simulink model "Simulation_18thJune"  (R2022b)
settings: Solver=VariableStepAuto  StartTime=0.0  StopTime=1.3  RelTol=1e-3
values from neighbouring files (symbols this model uses):
  C_f = 0.000112315*9    (= 0.001010835)    [Main.m]    (also in PSO_2paras.m = swarm(i,2); PSO_filter_2paras.m = swarm(i,2)/10000; Primary_test1.m; Script_18June.m = 0.0112315)
  f_c = 50e3    (= 50000)    [Main.m]    (also in Primary_test1.m; Script_18June.m; Script_23June.m; Script_5thJune.m)
  k = -0.5    [Main.m]    (also in Primary_test1.m; Savedata.m = 0.2909; Script_18June.m = 0.5; Script_23June.m)
  K_h11 = 0    [Main.m]    (also in PSO_HC.m = swarm(i,4); Primary_test1.m; Script_18June.m; Script_23June.m)
  K_h13 = 0    [Main.m]    (also in Primary_test1.m; Script_18June.m; Script_23June.m; Script_5thJune.m)
  K_h5 = 0    [Main.m]    (also in PSO_HC.m = swarm(i,1); Primary_test1.m = 1; Script_18June.m; Script_23June.m)
  K_h7 = 0    [Main.m]    (also in PSO_HC.m = swarm(i,2); Primary_test1.m; Script_18June.m; Script_23June.m)
  K_h9 = 0    [Main.m]    (also in PSO_HC.m = swarm(i,3); Script_18June.m; Script_23June.m; Script_5thJune.m)
  ki_pr = 160    [Main.m]    (also in PSO.m = swarm(i,2); Primary_test1.m; Savedata.m = 422.4716; Script_18June.m = 150)
  kL = 1e-7    (= 1e-07)    [Main.m]    (also in Primary_test1.m; Script_18June.m; Script_23June.m; Script_5thJune.m)
  Kp_pr = 1.7    [Main.m]    (also in PSO.m = swarm(i,1); Primary_test1.m; Savedata.m = 0.9028; Script_18June.m = 1)
  L_f = 0.000659829*1.4    (= 0.0009237606)    [Main.m]    (also in PSO_2paras.m = swarm(i,1); PSO_filter_2paras.m = swarm(i,1); Primary_test1.m; Script_18June.m = 0.000295603392)
  L_in1 = 0.35e-3    (= 0.00035)    [Main.m]    (also in Primary_test1.m; Script_18June.m; Script_23June.m; Script_5thJune.m)
  L_in2 = 0.35e-3    (= 0.00035)    [Main.m]    (also in Primary_test1.m; Script_18June.m; Script_23June.m; Script_5thJune.m)
  LD_ref1 = 100e-6    (= 0.0001)    [Main.m]    (also in Primary_test1.m; Script_18June.m = 5e-05; Script_23June.m = 1e-05; Script_5thJune.m = 1e-05)
  lo_co = 0.1    [Main.m]    (also in Primary_test1.m; Script_18June.m; Script_23June.m; Script_5thJune.m)
  load_off = 28    [Main.m]    (also in Primary_test1.m = 2; Script_18June.m; Script_23June.m; Script_5thJune.m = 10)
  load_on = 0.21    [Main.m]    (also in Primary_test1.m = 1; Script_18June.m; Script_23June.m; Script_5thJune.m)
  m_p1 = 9.4e-5/droopDivide    (= 9.4e-06)    [Main.m]    (also in Primary_test1.m; Script_18June.m = 9.4e-05; Script_23June.m = 9.4e-05; Script_5thJune.m = 5e-05)
  m_p2 = 9.4e-5/droopDivide    (= 9.4e-06)    [Main.m]    (also in Primary_test1.m; Script_18June.m = 9.4e-05; Script_23June.m = 9.4e-05; Script_5thJune.m = 5e-05)
  m_p3 = 11.4e-5/droopDivide    (= 1.14e-05)    [Main.m]    (also in Primary_test1.m; Script_18June.m = 0.000114; Script_23June.m = 0.000114; Script_5thJune.m = 6.42857142857e-05)
  m_p4 = 11.4e-5/droopDivide    (= 1.14e-05)    [Main.m]    (also in Primary_test1.m; Script_18June.m = 0.000114; Script_23June.m = 0.000114; Script_5thJune.m = 6.42857142857e-05)
  n_q1 = 1.3e-3/droopDivide2    (= 6.5e-05)    [Main.m]    (also in Primary_test1.m; Script_18June.m; Script_23June.m; Script_5thJune.m = 0.2)
  n_q2 = 1.3e-3/droopDivide2    (= 6.5e-05)    [Main.m]    (also in Primary_test1.m; Script_18June.m; Script_23June.m; Script_5thJune.m = 0.2)
  n_q3 = 1.5e-3/droopDivide2    (= 7.5e-05)    [Main.m]    (also in Primary_test1.m; Script_18June.m; Script_23June.m; Script_5thJune.m = 0.257142857143)
  n_q4 = 1.5e-3/droopDivide2    (= 7.5e-05)    [Main.m]    (also in Primary_test1.m; Script_18June.m; Script_23June.m; Script_5thJune.m = 0.257142857143)
  PMW = V_nom/0.55    [Main.m]    (also in Primary_test1.m; Script_18June.m = V_nom/0.4; Script_23June.m; Script_5thJune.m = 220*sqrt(2))
  R_f = 0.35    [Main.m]    (also in PSO_filter_2paras.m = 10*L_f; Primary_test1.m; Savedata.m = 0.249593207053; Script_18June.m = 0.1)
  R_in1 = 0.03    [Main.m]    (also in Primary_test1.m; Script_18June.m; Script_23June.m; Script_5thJune.m)
  R_in2 = 0.03    [Main.m]    (also in Primary_test1.m; Script_18June.m; Script_23June.m; Script_5thJune.m)
  Ts = 10e-6    (= 1e-05)    [Main.m]    (also in Primary_test1.m; Script_18June.m; Script_23June.m; Script_5thJune.m)
  V_nom = 220*sqrt(2)    [Main.m]    (also in Primary_test1.m; Script_18June.m; Script_23June.m; Script_5thJune.m)
  Vdc = 600    [Main.m]    (also in Primary_test1.m; Script_18June.m; Script_23June.m; Script_5thJune.m)
  w_c_high = 2*pi*50    (= 314.159265359)    [Main.m]    (also in Primary_test1.m; Script_18June.m = 307.876080052; Script_23June.m; Script_5thJune.m = 307.876080052)
  w_nom = 2*pi*f    (= 314.159265359)    [Main.m]    (also in Primary_test1.m; Script_18June.m; Script_23June.m; Script_5thJune.m)
  wc_hc = 1    [Main.m]    (also in Primary_test1.m; Script_18June.m = 0.3; Script_23June.m; Script_5thJune.m = 0.3)
  wc_pr = 3    [Main.m]    (also in PSO.m = swarm(i,3); Primary_test1.m; Savedata.m = 1.36672; Script_18June.m = 1.5)
undefined symbols (not defined in the file or in its folder): i
libraries: eeGeneralControl x16, spsThreePhaseSeriesRLCBranchLib x15, spsThreePhaseVIMeasurementLib x12, spsabctodq0Lib x12, slpidlib x8, spsThreePhaseSeriesRLCLoadLib x5, spsThreePhaseBreakerLib x5, spsDCVoltageSourceLib x5, spsSeriesRLCBranchLib x5, spsTriangleGeneratorLib x4, spsTwoLevelConverterLib x4, spsIGBTLib x2
(part 3 of 4)

== system Simulation_18thJune/Voltage Source Inverter 2/PLL_1p2 ==
  v : Inport
  2pi : Constant  Value=2*pi
  Low-Pass Filter (Discrete or Continuous) : eeGeneralControl/Low-Pass Filter (Discrete or Continuous)  K=1  T=lo_co  B=inf  A=-inf  init_option=Inherited from block input  x0=0  Ts=-1
  PID Controller : slpidlib/PID Controller  Controller=PI  Form=Parallel  TimeDomain=Continuous-time  UseExternalTs=off  SampleTime=-1  IntegratorMethod=Forward Euler  FilterMethod=Forward Euler  ControllerParametersSource=internal  P=100.15925  I=9869  UseKiTs=off  D=0  N=100  UseFilter=on  TunerSelectOption=Transfer Function Based (PID Tuner App)  InitialConditionSource=internal  InitialConditionForIntegrator=0  InitialConditionForFilter=0  DifferentiatorICPrevScaledInput=0  ExternalReset=none  TrackingMode=off  Kt=1  LimitOutput=off  SatLimitsSource=internal  UpperSaturationLimit=inf  LowerSaturationLimit=-inf  LinearizeAsGain=off  AntiWindupMode=none  Kb=1  LimitIntegrator=off  UpperIntegratorSaturationLimit=inf  LowerIntegratorSaturationLimit=-inf  POutMin=[]  POutMax=[]  IOutMin=[]  IOutMax=[]  DOutMin=[]  DOutMax=[]  NOutMin=[]  NOutMax=[]  SumOutMin=[]  SumOutMax=[]  SaturationOutMin=[]  SaturationOutMax=[]  PParamMin=[]  PParamMax=[]  IParamMin=[]  IParamMax=[]  DParamMin=[]  DParamMax=[]  NParamMin=[]  NParamMax=[]  KbParamMin=[]  KbParamMax=[]  KtParamMin=[]  KtParamMax=[]  KbOutMin=[]  KbOutMax=[]  KtOutMin=[]  KtOutMax=[]  IntegratorOutMin=[]  IntegratorOutMax=[]  FilterOutMin=[]  FilterOutMax=[]  SumI1OutMin=[]  SumI1OutMax=[]  SumI2OutMin=[]  SumI2OutMax=[]  SumI3OutMin=[]  SumI3OutMax=[]  SumI4OutMin=[]  SumI4OutMax=[]  SumDOutMin=[]  SumDOutMax=[]  DifferentiatorOutMin=[]  DifferentiatorOutMax=[]  FilterDiffOutCoefMin=[]  FilterDiffOutCoefMax=[]  ReciprocalOutMin=[]  ReciprocalOutMax=[]  SumDenOutMin=[]  SumDenOutMax=[]  SumNumOutMin=[]  SumNumOutMax=[]  DivideOutMin=[]  DivideOutMax=[]  UdiffTsProdOutMin=[]  UdiffTsProdOutMax=[]  NTsProdOutMin=[]  NTsProdOutMax=[]  UintegralTsProdOutMin=[]  UintegralTsProdOutMax=[]  UngainTsProdOutMin=[]  UngainTsProdOutMax=[]  ClampingZeroOutDataTypeStr=Inherit: Inherit via back propagation  ClampingZeroOutMin=[]  ClampingZeroOutMax=[]  FilterDenConstantOutDataTypeStr=Inherit: Inherit via back propagation  FilterDenConstantOutMin=[]  FilterDenConstantOutMax=[]  PCopyOutDataTypeStr=Inherit: Inherit via back propagation  PCopyOutMin=[]  PCopyOutMax=[]  NCopyOutDataTypeStr=Inherit: Inherit via back propagation  NCopyOutMin=[]  NCopyOutMax=[]  IntegratorContinuousStateAttributes=''  IntegratorStateMustResolveToSignalObject=off  IntegratorRTWStateStorageClass=Auto  FilterContinuousStateAttributes=''  FilterStateMustResolveToSignalObject=off  FilterRTWStateStorageClass=Auto  ParallelPVariant=InternalParameters  IdealPVariant=Disabled  IVariant=InternalParameters  DVariant=Disabled  IntegratorVariant=Continuous  SatVariant=Disabled  AWVariant=Passthrough  PCopyVariant=Disabled  TRVariant=Disabled  FdbkBlocksVariant=Forward  IdealPFdbkVariant=Disabled  SatFdbkVariant=Disabled  DerivativeFilterVariant=Disabled  NVariant=Disabled  NCopyVariant=Disabled_SignalSpec  FilterICVariant=Disabled  IntegratorICVariant=InternalICs  ExternalResetVariant=Disabled  TRSumVariant=Passthrough  SumFdbkVariant=Disabled  SumVariant=Sum_PI  TsampFilterVariant=InternalTs  TsampNgainVariant=Passthrough  TsampIntegralVariant=Passthrough  ExternalSaturationOutDataTypeStr=Inherit: Same as second input
  Reset1 : RelationalOperator  OutDataTypeStr=boolean  InputSameDT=off
  Scope : Scope
  Sqrt : Sqrt
  Square : Math  Operator=square
  Square1 : Math  Operator=square
  Sum : Sum  Inputs=|++
  Sum1 : Sum  Inputs=|++
  TienXuly : Subsystem  mask{k=0.5, fc1=50, fc2=10}
      mask prompts: k "he so k"; fc1 "Tan so cat cua bo loc bac 2"; fc2 "Tan so cat cua bo loc thong thap"
  Tinhtheta : Integrator  ExternalReset=rising  UpperSaturationLimit=2*pi
  apha-beta=>dq : Subsystem
  wff : Constant  Value=50*2*pi
  v_dq : Outport
  omega : Outport  Port=2
  wires:
  PID Controller/1 -> Sum1/1
  v/1 -> TienXuly/1(v)
  Tinhtheta/1 -> apha-beta=>dq/1(Theta), Reset1/1
  TienXuly/2(v'q) -> apha-beta=>dq/3(Ubeta)
  apha-beta=>dq/1(vq) -> Square1/1, PID Controller/1
  TienXuly/1(v') -> apha-beta=>dq/2(Uapha)
  2pi/1 -> Reset1/2
  wff/1 -> Sum1/2
  Reset1/1 -> Tinhtheta/2
  apha-beta=>dq/2(vd) -> Square/1
  Square/1 -> Sum/1
  Square1/1 -> Sum/2
  Sum/1 -> Sqrt/1
  Sqrt/1 -> v_dq/1
  Sum1/1 -> Low-Pass Filter (Discrete or Continuous)/1, Tinhtheta/1  "P"
  Low-Pass Filter (Discrete or Continuous)/1 -> Scope/1, omega/1  "P"

== system Simulation_18thJune/Voltage Source Inverter 2/PMW ==
  REF : Inport
  Tri_signal : Inport  Port=2
  Demux : Demux  Outputs=3
  Mux : Mux  Inputs=6
  NOT : Logic  Operator=NOT  AllPortsSameDT=off  OutDataTypeStr=boolean
  NOT1 : Logic  Operator=NOT  AllPortsSameDT=off  OutDataTypeStr=boolean
  NOT2 : Logic  Operator=NOT  AllPortsSameDT=off  OutDataTypeStr=boolean
  Relational Operator : RelationalOperator  OutDataTypeStr=boolean  RndMeth=Simplest  InputSameDT=off
  Relational Operator1 : RelationalOperator  OutDataTypeStr=boolean  RndMeth=Simplest  InputSameDT=off
  Relational Operator2 : RelationalOperator  OutDataTypeStr=boolean  RndMeth=Simplest  InputSameDT=off
  Scope : Scope
  Scope1 : Scope
  Scope2 : Scope  NumInputPorts=2
  Out1 : Outport
  wires:
  Demux/1 -> Relational Operator/1
  Tri_signal/1 -> Relational Operator1/2, Relational Operator/2, Relational Operator2/2
  Demux/2 -> Relational Operator1/1
  Demux/3 -> Relational Operator2/1
  REF/1 -> Scope1/1, Demux/1
  Relational Operator/1 -> Scope2/1, Mux/1, NOT/1
  NOT/1 -> Scope2/2, Mux/2
  Relational Operator1/1 -> NOT1/1, Mux/3
  NOT1/1 -> Mux/4
  Relational Operator2/1 -> Mux/5, NOT2/1
  NOT2/1 -> Mux/6
  Mux/1 -> Scope/1, Out1/1

== system Simulation_18thJune/Voltage Source Inverter 2/PQ calculator ==
  Vod : Inport
  Voq : Inport  Port=2
  Iod : Inport  Port=3
  Ioq : Inport  Port=4
  Product{,1..3} (4 alike) : Product
  Scope : Scope
  Sum10 : Sum  Inputs=|++
  Sum11 : Sum  Inputs=|+-
  p_hat : Outport
  q_hat : Outport  Port=2
  wires:
  Product3/1 -> Sum11/2
  Product1/1 -> Sum10/2
  Voq/1 -> Product3/1, Product1/1
  Iod/1 -> Product/2, Product3/2
  Product2/1 -> Sum11/1
  Ioq/1 -> Product1/2, Product2/2
  Product/1 -> Sum10/1
  Vod/1 -> Scope/1, Product/1, Product2/1
  Sum11/1 -> q_hat/1  "q_hat"
  Sum10/1 -> p_hat/1  "p_hat"

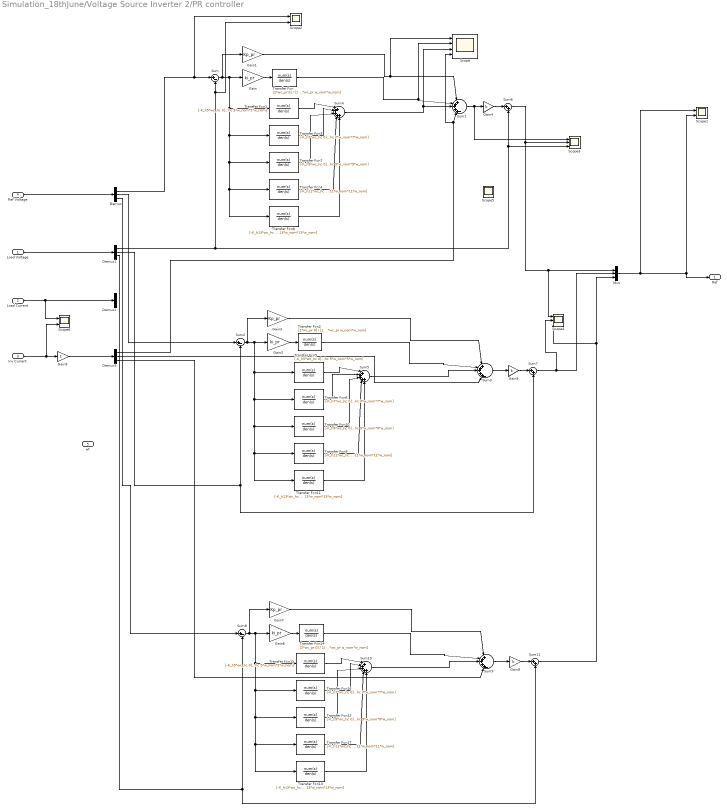
== system Simulation_18thJune/Voltage Source Inverter 2/PR controller ==
  Load Voltage : Inport
  Load Current : Inport  Port=2
  Inv Current : Inport  Port=3
  Ref Voltage : Inport  Port=4
  wt : Inport  Port=5
  Demux{,1..3} (4 alike) : Demux  Outputs=3
  Gain : Gain  Gain=ki_pr
  Gain1 : Gain  Gain=Kp_pr
  Gain2 : Gain  Gain=ki_pr
  Gain3 : Gain  Gain=Kp_pr
  Gain4 : Gain  Gain=k
  Gain5 : Gain  Gain=k
  Gain6 : Gain  Gain=ki_pr
  Gain7 : Gain  Gain=Kp_pr
  Gain8 : Gain  Gain=k
  Gain9 : Gain
  Mux : Mux  Inputs=3
  Scope : Scope  NumInputPorts=4
  Scope{1..2,5..6} (4 alike) : Scope  NumInputPorts=2
  Scope3 : Scope  NumInputPorts=3
  Scope4 : Scope  NumInputPorts=3
  Sum : Sum  Inputs=|+-
  Sum1 : Sum  Inputs=|+++++-
  Sum10 : Sum  Inputs=|+++++
  Sum11 : Sum  Inputs=|++
  Sum2 : Sum  Inputs=|+-
  Sum3 : Sum  Inputs=|+++++-
  Sum4 : Sum  Inputs=|+++++
  Sum5 : Sum  Inputs=|+++++
  Sum6 : Sum  Inputs=|++
  Sum7 : Sum  Inputs=|++
  Sum8 : Sum  Inputs=|+-
  Sum9 : Sum  Inputs=|+++++-
  Transfer Fcn : TransferFcn  Numerator=[2*wc_pr 0]  Denominator=[1 2*wc_pr*wc_pr w_nom*w_nom]
  Transfer Fcn1 : TransferFcn  Numerator=[-K_h5*wc_hc 0]  Denominator=[1 2*wc_hc 5*w_nom*5*w_nom]
  Transfer Fcn10 : TransferFcn  Numerator=[-K_h9*wc_hc 0]  Denominator=[1 2*wc_hc 9*w_nom*9*w_nom]
  Transfer Fcn11 : TransferFcn  Numerator=[-K_h13*wc_hc 0]  Denominator=[1 2*wc_hc 13*w_nom*13*w_nom]
  Transfer Fcn12 : TransferFcn  Numerator=[-K_h9*wc_hc 0]  Denominator=[1 2*wc_hc 9*w_nom*9*w_nom]
  Transfer Fcn13 : TransferFcn  Numerator=[-K_h13*wc_hc 0]  Denominator=[1 2*wc_hc 13*w_nom*13*w_nom]
  Transfer Fcn14 : TransferFcn  Numerator=[2*wc_pr 0]  Denominator=[1 2*wc_pr*wc_pr w_nom*w_nom]
  Transfer Fcn15 : TransferFcn  Numerator=[-K_h5*wc_hc 0]  Denominator=[1 2*wc_hc 5*w_nom*5*w_nom]
  Transfer Fcn16 : TransferFcn  Numerator=[-K_h7*wc_hc 0]  Denominator=[1 2*wc_hc 7*w_nom*7*w_nom]
  Transfer Fcn17 : TransferFcn  Numerator=[-K_h11*wc_hc 0]  Denominator=[1 2*wc_hc 11*w_nom*11*w_nom]
  Transfer Fcn2 : TransferFcn  Numerator=[2*wc_pr 0]  Denominator=[1 2*wc_pr*wc_pr w_nom*w_nom]
  Transfer Fcn3 : TransferFcn  Numerator=[-K_h7*wc_hc 0]  Denominator=[1 2*wc_hc 7*w_nom*7*w_nom]
  Transfer Fcn4 : TransferFcn  Numerator=[-K_h11*wc_hc 0]  Denominator=[1 2*wc_hc 11*w_nom*11*w_nom]
  Transfer Fcn5 : TransferFcn  Numerator=[-K_h5*wc_hc 0]  Denominator=[1 2*wc_hc 5*w_nom*5*w_nom]
  Transfer Fcn6 : TransferFcn  Numerator=[-K_h7*wc_hc 0]  Denominator=[1 2*wc_hc 7*w_nom*7*w_nom]
  Transfer Fcn7 : TransferFcn  Numerator=[-K_h9*wc_hc 0]  Denominator=[1 2*wc_hc 9*w_nom*9*w_nom]
  Transfer Fcn8 : TransferFcn  Numerator=[-K_h13*wc_hc 0]  Denominator=[1 2*wc_hc 13*w_nom*13*w_nom]
  Transfer Fcn9 : TransferFcn  Numerator=[-K_h11*wc_hc 0]  Denominator=[1 2*wc_hc 11*w_nom*11*w_nom]
  Ref : Outport
  wires:
  Ref Voltage/1 -> Demux/1
  Sum/1 -> Gain1/1, Transfer Fcn8/1, Transfer Fcn4/1, Transfer Fcn7/1, Transfer Fcn3/1, Transfer Fcn1/1, Gain/1
  Gain/1 -> Transfer Fcn/1
  Gain1/1 -> Scope/1, Sum1/1
  Transfer Fcn/1 -> Scope/2, Sum1/2
  Mux/1 -> Ref/1, Scope1/2, Scope1/1
  Sum4/1 -> Scope/3, Sum1/3
  Transfer Fcn1/1 -> Sum4/1
  Transfer Fcn3/1 -> Sum4/2
  Transfer Fcn7/1 -> Sum4/3
  Transfer Fcn4/1 -> Sum4/4
  Transfer Fcn8/1 -> Sum4/5
  Load Voltage/1 -> Demux1/1
  Inv Current/1 -> Scope6/2, Gain9/1
  Demux/1 -> Scope2/1, Sum/1
  Demux1/1 -> Sum6/2, Scope3/3, Scope2/2, Sum/2
  Demux3/1 -> Scope/4, Sum1/5
  Sum1/1 -> Scope3/1, Gain4/1
  Gain4/1 -> Sum6/1
  Sum6/1 -> Scope4/1, Mux/1, Scope3/2
  Demux1/2 -> Sum7/2, Sum2/2
  Transfer Fcn9/1 -> Sum5/4
  Sum5/1 -> Sum3/3
  Transfer Fcn6/1 -> Sum5/2
  Transfer Fcn5/1 -> Sum5/1
  Transfer Fcn11/1 -> Sum5/5
  Transfer Fcn10/1 -> Sum5/3
  Gain5/1 -> Sum7/1
  Gain3/1 -> Sum3/1
  Demux/2 -> Sum2/1
  Sum3/1 -> Gain5/1
  Sum2/1 -> Gain3/1, Transfer Fcn11/1, Transfer Fcn9/1, Transfer Fcn10/1, Transfer Fcn6/1, Transfer Fcn5/1, Gain2/1
  Transfer Fcn2/1 -> Sum3/2
  Gain2/1 -> Transfer Fcn2/1
  Sum7/1 -> Scope4/2, Mux/2
  Demux1/3 -> Sum11/2, Sum8/2
  Gain6/1 -> Transfer Fcn14/1
  Sum8/1 -> Gain7/1, Transfer Fcn13/1, Transfer Fcn17/1, Transfer Fcn12/1, Transfer Fcn16/1, Transfer Fcn15/1, Gain6/1
  Gain8/1 -> Sum11/1
  Sum9/1 -> Gain8/1
  Transfer Fcn13/1 -> Sum10/5
  Transfer Fcn12/1 -> Sum10/3
  Gain7/1 -> Sum9/1
  Transfer Fcn15/1 -> Sum10/1
  Transfer Fcn16/1 -> Sum10/2
  Transfer Fcn17/1 -> Sum10/4
  Sum11/1 -> Scope4/3, Mux/3
  Sum10/1 -> Sum9/3
  Demux/3 -> Sum8/1
  Transfer Fcn14/1 -> Sum9/2
  Demux3/2 -> Sum3/5
  Demux3/3 -> Sum9/5
  Load Current/1 -> Scope6/1, Demux2/1
  Gain9/1 -> Demux3/1

== system Simulation_18thJune/Voltage Source Inverter 2/THD measurement ==
  In1 : Inport
  Demux : Demux  Outputs=3
  To Workspace : ToWorkspace  VariableName=phase1  SaveFormat=Structure With Time  SampleTime=-1
  To Workspace1 : ToWorkspace  VariableName=phase2  SaveFormat=Structure With Time  SampleTime=-1
  To Workspace2 : ToWorkspace  VariableName=phase3  SaveFormat=Structure With Time  SampleTime=-1
  wires:
  In1/1 -> Demux/1
  Demux/1 -> To Workspace/1
  Demux/2 -> To Workspace1/1
  Demux/3 -> To Workspace2/1

== system Simulation_18thJune/Voltage Source Inverter 2/dq converter ==
  Vodq : Inport
  Iodq : Inport  Port=2
  Ildq : Inport  Port=3
  wt : Inport  Port=4
  Scope : Scope
  Scope1 : Scope
  Subsystem : Subsystem
  Subsystem1 : Subsystem
  Subsystem2 : Subsystem
  Vod : Outport
  Voq : Outport  Port=2
  Iod : Outport  Port=3
  Ioq : Outport  Port=4
  Ild : Outport  Port=5
  Ilq : Outport  Port=6
  wires:
  Subsystem/1(Out1) -> Scope/1, Vod/1  "Vod"
  Subsystem1/1(Out1) -> Iod/1  "Iod"
  Subsystem/2(Out2) -> Voq/1  "Voq"
  wt/1 -> Subsystem2/2(wt), Subsystem1/2(wt), Subsystem/2(wt)
  Subsystem1/2(Out2) -> Ioq/1  "Ioq"
  Iodq/1 -> Subsystem1/1(abc)
  Subsystem2/2(Out2) -> Ilq/1  "Ilq"
  Ildq/1 -> Subsystem2/1(abc)
  Vodq/1 -> Subsystem/1(abc)
  Subsystem2/1(Out1) -> Scope1/1, Ild/1  "Vod"

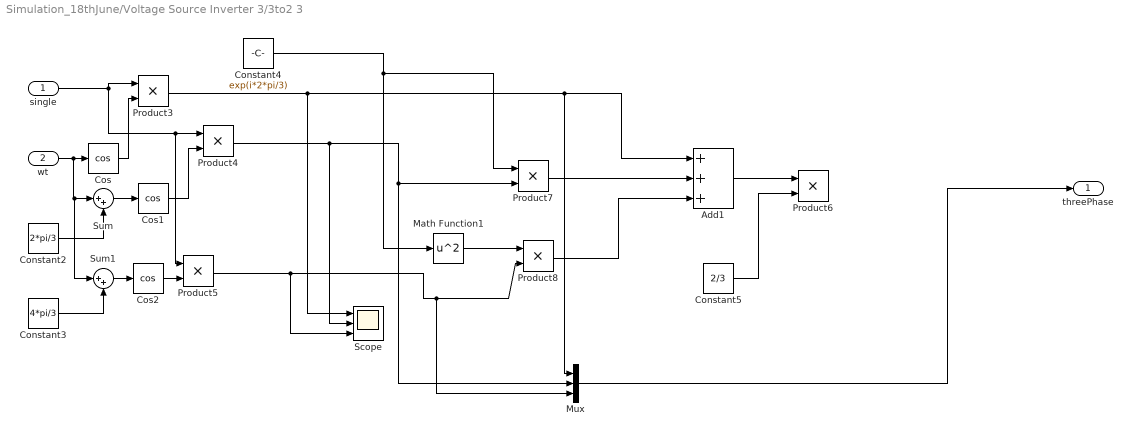
== system Simulation_18thJune/Voltage Source Inverter 3/3to2 3 ==
  "single " : Inport
  "wt " : Inport  Port=2
  Add1 : Sum  Inputs=+++
  Constant2 : Constant  Value=2*pi/3
  Constant3 : Constant  Value=4*pi/3
  Constant4 : Constant  Value=exp(i*2*pi/3)
  Constant5 : Constant  Value=2/3
  Cos : Trigonometry  Operator=cos
  Cos1 : Trigonometry  Operator=cos
  Cos2 : Trigonometry  Operator=cos
  Math Function1 : Math  Operator=square  SignedPower=on
  Mux : Mux  Inputs=3
  Product{3..8} (6 alike) : Product  RndMeth=Zero
  Scope : Scope  NumInputPorts=3
  Sum : Sum  Inputs=|++
  Sum1 : Sum  Inputs=|++
  threePhase : Outport  VectorParamsAs1DForOutWhenUnconnected=off
  wires:
  "single "/1 -> Product5/1, Product4/1, Product3/1
  Cos/1 -> Product3/2
  Constant2/1 -> Sum/2
  Sum/1 -> Cos1/1
  Cos1/1 -> Product4/2
  "wt "/1 -> Sum1/1, Sum/1, Cos/1
  Constant3/1 -> Sum1/2
  Sum1/1 -> Cos2/1
  Cos2/1 -> Product5/2
  Constant4/1 -> Product7/1, Math Function1/1
  Product7/1 -> Add1/2
  Add1/1 -> Product6/1
  Product8/1 -> Add1/3
  Product5/1 -> Scope/3, Mux/3, Product8/2
  Product3/1 -> Scope/1, Mux/1, Add1/1
  Constant5/1 -> Product6/2
  Product4/1 -> Scope/2, Mux/2, Product7/2
  Math Function1/1 -> Product8/1
  Mux/1 -> threePhase/1

== system Simulation_18thJune/Voltage Source Inverter 3/Droop for secondary control2 ==
  P : Inport
  w_nom : Inport  Port=2
  V_nom : Inport  Port=3
  Q : Inport  Port=4
  Gain4 : Gain  Gain=n_q
  Gain5 : Gain  Gain=m_p
  Integrator : Integrator  WrapState=on  WrappedStateUpperValue=2*pi  WrappedStateLowerValue=0
  Sum1 : Sum  Inputs=|+-
  Sum2 : Sum  Inputs=|+-
  Vref : Outport
  wt : Outport  Port=2
  wo : Outport  Port=3
  wires:
  P/1 -> Gain5/1
  w_nom/1 -> Sum2/1
  Gain5/1 -> Sum2/2
  Sum2/1 -> wo/1, Integrator/1  "w"
  Integrator/1 -> wt/1
  V_nom/1 -> Sum1/1  "Vod_s"
  Gain4/1 -> Sum1/2
  Q/1 -> Gain4/1
  Sum1/1 -> Vref/1  "Vod_s"

== system Simulation_18thJune/Voltage Source Inverter 3/Low-pass filter ==
  p_hat : Inport
  q_hat : Inport  Port=2
  Low-Pass Filter (Discrete or Continuous) : eeGeneralControl/Low-Pass Filter (Discrete or Continuous)  K=1  T=lo_co  B=inf  A=-inf  init_option=Inherited from block input  x0=0  Ts=-1
  Low-Pass Filter (Discrete or Continuous)1 : eeGeneralControl/Low-Pass Filter (Discrete or Continuous)  K=1  T=lo_co  B=inf  A=-inf  init_option=Inherited from block input  x0=0  Ts=-1
  P : Outport
  Q : Outport  Port=2
  wires:
  q_hat/1 -> Low-Pass Filter (Discrete or Continuous)1/1
  Low-Pass Filter (Discrete or Continuous)1/1 -> Q/1  "Q"
  Low-Pass Filter (Discrete or Continuous)/1 -> P/1  "P"
  p_hat/1 -> Low-Pass Filter (Discrete or Continuous)/1

== system Simulation_18thJune/Voltage Source Inverter 3/PLL_1p1 ==
  v : Inport
  2pi : Constant  Value=2*pi
  Low-Pass Filter (Discrete or Continuous) : eeGeneralControl/Low-Pass Filter (Discrete or Continuous)  K=1  T=lo_co  B=inf  A=-inf  init_option=Inherited from block input  x0=0  Ts=-1
  PID Controller : slpidlib/PID Controller  Controller=PI  Form=Parallel  TimeDomain=Continuous-time  UseExternalTs=off  SampleTime=-1  IntegratorMethod=Forward Euler  FilterMethod=Forward Euler  ControllerParametersSource=internal  P=100.15925  I=9869  UseKiTs=off  D=0  N=100  UseFilter=on  TunerSelectOption=Transfer Function Based (PID Tuner App)  InitialConditionSource=internal  InitialConditionForIntegrator=0  InitialConditionForFilter=0  DifferentiatorICPrevScaledInput=0  ExternalReset=none  TrackingMode=off  Kt=1  LimitOutput=off  SatLimitsSource=internal  UpperSaturationLimit=inf  LowerSaturationLimit=-inf  LinearizeAsGain=off  AntiWindupMode=none  Kb=1  LimitIntegrator=off  UpperIntegratorSaturationLimit=inf  LowerIntegratorSaturationLimit=-inf  POutMin=[]  POutMax=[]  IOutMin=[]  IOutMax=[]  DOutMin=[]  DOutMax=[]  NOutMin=[]  NOutMax=[]  SumOutMin=[]  SumOutMax=[]  SaturationOutMin=[]  SaturationOutMax=[]  PParamMin=[]  PParamMax=[]  IParamMin=[]  IParamMax=[]  DParamMin=[]  DParamMax=[]  NParamMin=[]  NParamMax=[]  KbParamMin=[]  KbParamMax=[]  KtParamMin=[]  KtParamMax=[]  KbOutMin=[]  KbOutMax=[]  KtOutMin=[]  KtOutMax=[]  IntegratorOutMin=[]  IntegratorOutMax=[]  FilterOutMin=[]  FilterOutMax=[]  SumI1OutMin=[]  SumI1OutMax=[]  SumI2OutMin=[]  SumI2OutMax=[]  SumI3OutMin=[]  SumI3OutMax=[]  SumI4OutMin=[]  SumI4OutMax=[]  SumDOutMin=[]  SumDOutMax=[]  DifferentiatorOutMin=[]  DifferentiatorOutMax=[]  FilterDiffOutCoefMin=[]  FilterDiffOutCoefMax=[]  ReciprocalOutMin=[]  ReciprocalOutMax=[]  SumDenOutMin=[]  SumDenOutMax=[]  SumNumOutMin=[]  SumNumOutMax=[]  DivideOutMin=[]  DivideOutMax=[]  UdiffTsProdOutMin=[]  UdiffTsProdOutMax=[]  NTsProdOutMin=[]  NTsProdOutMax=[]  UintegralTsProdOutMin=[]  UintegralTsProdOutMax=[]  UngainTsProdOutMin=[]  UngainTsProdOutMax=[]  ClampingZeroOutDataTypeStr=Inherit: Inherit via back propagation  ClampingZeroOutMin=[]  ClampingZeroOutMax=[]  FilterDenConstantOutDataTypeStr=Inherit: Inherit via back propagation  FilterDenConstantOutMin=[]  FilterDenConstantOutMax=[]  PCopyOutDataTypeStr=Inherit: Inherit via back propagation  PCopyOutMin=[]  PCopyOutMax=[]  NCopyOutDataTypeStr=Inherit: Inherit via back propagation  NCopyOutMin=[]  NCopyOutMax=[]  IntegratorContinuousStateAttributes=''  IntegratorStateMustResolveToSignalObject=off  IntegratorRTWStateStorageClass=Auto  FilterContinuousStateAttributes=''  FilterStateMustResolveToSignalObject=off  FilterRTWStateStorageClass=Auto  ParallelPVariant=InternalParameters  IdealPVariant=Disabled  IVariant=InternalParameters  DVariant=Disabled  IntegratorVariant=Continuous  SatVariant=Disabled  AWVariant=Passthrough  PCopyVariant=Disabled  TRVariant=Disabled  FdbkBlocksVariant=Forward  IdealPFdbkVariant=Disabled  SatFdbkVariant=Disabled  DerivativeFilterVariant=Disabled  NVariant=Disabled  NCopyVariant=Disabled_SignalSpec  FilterICVariant=Disabled  IntegratorICVariant=InternalICs  ExternalResetVariant=Disabled  TRSumVariant=Passthrough  SumFdbkVariant=Disabled  SumVariant=Sum_PI  TsampFilterVariant=InternalTs  TsampNgainVariant=Passthrough  TsampIntegralVariant=Passthrough  ExternalSaturationOutDataTypeStr=Inherit: Same as second input
  Reset1 : RelationalOperator  OutDataTypeStr=boolean  InputSameDT=off
  Scope : Scope
  Sqrt : Sqrt
  Square : Math  Operator=square
  Square1 : Math  Operator=square
  Sum : Sum  Inputs=|++
  Sum1 : Sum  Inputs=|++
  TienXuly : Subsystem  mask{k=0.5, fc1=50, fc2=10}
      mask prompts: k "he so k"; fc1 "Tan so cat cua bo loc bac 2"; fc2 "Tan so cat cua bo loc thong thap"
  Tinhtheta : Integrator  ExternalReset=rising  UpperSaturationLimit=2*pi
  apha-beta=>dq : Subsystem
  wff : Constant  Value=50*2*pi
  v_dq : Outport
  omega : Outport  Port=2
  wires:
  PID Controller/1 -> Sum1/1
  v/1 -> TienXuly/1(v)
  Tinhtheta/1 -> apha-beta=>dq/1(Theta), Reset1/1
  TienXuly/2(v'q) -> apha-beta=>dq/3(Ubeta)
  apha-beta=>dq/1(vq) -> Square1/1, PID Controller/1
  TienXuly/1(v') -> apha-beta=>dq/2(Uapha)
  2pi/1 -> Reset1/2
  wff/1 -> Sum1/2
  Reset1/1 -> Tinhtheta/2
  apha-beta=>dq/2(vd) -> Square/1
  Square/1 -> Sum/1
  Square1/1 -> Sum/2
  Sum/1 -> Sqrt/1
  Sqrt/1 -> v_dq/1
  Sum1/1 -> Low-Pass Filter (Discrete or Continuous)/1, Tinhtheta/1  "P"
  Low-Pass Filter (Discrete or Continuous)/1 -> Scope/1, omega/1  "P"

== system Simulation_18thJune/Voltage Source Inverter 3/PLL_1p2 ==
  v : Inport
  2pi : Constant  Value=2*pi
  Low-Pass Filter (Discrete or Continuous) : eeGeneralControl/Low-Pass Filter (Discrete or Continuous)  K=1  T=lo_co  B=inf  A=-inf  init_option=Inherited from block input  x0=0  Ts=-1
  PID Controller : slpidlib/PID Controller  Controller=PI  Form=Parallel  TimeDomain=Continuous-time  UseExternalTs=off  SampleTime=-1  IntegratorMethod=Forward Euler  FilterMethod=Forward Euler  ControllerParametersSource=internal  P=100.15925  I=9869  UseKiTs=off  D=0  N=100  UseFilter=on  TunerSelectOption=Transfer Function Based (PID Tuner App)  InitialConditionSource=internal  InitialConditionForIntegrator=0  InitialConditionForFilter=0  DifferentiatorICPrevScaledInput=0  ExternalReset=none  TrackingMode=off  Kt=1  LimitOutput=off  SatLimitsSource=internal  UpperSaturationLimit=inf  LowerSaturationLimit=-inf  LinearizeAsGain=off  AntiWindupMode=none  Kb=1  LimitIntegrator=off  UpperIntegratorSaturationLimit=inf  LowerIntegratorSaturationLimit=-inf  POutMin=[]  POutMax=[]  IOutMin=[]  IOutMax=[]  DOutMin=[]  DOutMax=[]  NOutMin=[]  NOutMax=[]  SumOutMin=[]  SumOutMax=[]  SaturationOutMin=[]  SaturationOutMax=[]  PParamMin=[]  PParamMax=[]  IParamMin=[]  IParamMax=[]  DParamMin=[]  DParamMax=[]  NParamMin=[]  NParamMax=[]  KbParamMin=[]  KbParamMax=[]  KtParamMin=[]  KtParamMax=[]  KbOutMin=[]  KbOutMax=[]  KtOutMin=[]  KtOutMax=[]  IntegratorOutMin=[]  IntegratorOutMax=[]  FilterOutMin=[]  FilterOutMax=[]  SumI1OutMin=[]  SumI1OutMax=[]  SumI2OutMin=[]  SumI2OutMax=[]  SumI3OutMin=[]  SumI3OutMax=[]  SumI4OutMin=[]  SumI4OutMax=[]  SumDOutMin=[]  SumDOutMax=[]  DifferentiatorOutMin=[]  DifferentiatorOutMax=[]  FilterDiffOutCoefMin=[]  FilterDiffOutCoefMax=[]  ReciprocalOutMin=[]  ReciprocalOutMax=[]  SumDenOutMin=[]  SumDenOutMax=[]  SumNumOutMin=[]  SumNumOutMax=[]  DivideOutMin=[]  DivideOutMax=[]  UdiffTsProdOutMin=[]  UdiffTsProdOutMax=[]  NTsProdOutMin=[]  NTsProdOutMax=[]  UintegralTsProdOutMin=[]  UintegralTsProdOutMax=[]  UngainTsProdOutMin=[]  UngainTsProdOutMax=[]  ClampingZeroOutDataTypeStr=Inherit: Inherit via back propagation  ClampingZeroOutMin=[]  ClampingZeroOutMax=[]  FilterDenConstantOutDataTypeStr=Inherit: Inherit via back propagation  FilterDenConstantOutMin=[]  FilterDenConstantOutMax=[]  PCopyOutDataTypeStr=Inherit: Inherit via back propagation  PCopyOutMin=[]  PCopyOutMax=[]  NCopyOutDataTypeStr=Inherit: Inherit via back propagation  NCopyOutMin=[]  NCopyOutMax=[]  IntegratorContinuousStateAttributes=''  IntegratorStateMustResolveToSignalObject=off  IntegratorRTWStateStorageClass=Auto  FilterContinuousStateAttributes=''  FilterStateMustResolveToSignalObject=off  FilterRTWStateStorageClass=Auto  ParallelPVariant=InternalParameters  IdealPVariant=Disabled  IVariant=InternalParameters  DVariant=Disabled  IntegratorVariant=Continuous  SatVariant=Disabled  AWVariant=Passthrough  PCopyVariant=Disabled  TRVariant=Disabled  FdbkBlocksVariant=Forward  IdealPFdbkVariant=Disabled  SatFdbkVariant=Disabled  DerivativeFilterVariant=Disabled  NVariant=Disabled  NCopyVariant=Disabled_SignalSpec  FilterICVariant=Disabled  IntegratorICVariant=InternalICs  ExternalResetVariant=Disabled  TRSumVariant=Passthrough  SumFdbkVariant=Disabled  SumVariant=Sum_PI  TsampFilterVariant=InternalTs  TsampNgainVariant=Passthrough  TsampIntegralVariant=Passthrough  ExternalSaturationOutDataTypeStr=Inherit: Same as second input
  Reset1 : RelationalOperator  OutDataTypeStr=boolean  InputSameDT=off
  Scope : Scope
  Sqrt : Sqrt
  Square : Math  Operator=square
  Square1 : Math  Operator=square
  Sum : Sum  Inputs=|++
  Sum1 : Sum  Inputs=|++
  TienXuly : Subsystem  mask{k=0.5, fc1=50, fc2=10}
      mask prompts: k "he so k"; fc1 "Tan so cat cua bo loc bac 2"; fc2 "Tan so cat cua bo loc thong thap"
  Tinhtheta : Integrator  ExternalReset=rising  UpperSaturationLimit=2*pi
  apha-beta=>dq : Subsystem
  wff : Constant  Value=50*2*pi
  v_dq : Outport
  omega : Outport  Port=2
  wires:
  PID Controller/1 -> Sum1/1
  v/1 -> TienXuly/1(v)
  Tinhtheta/1 -> apha-beta=>dq/1(Theta), Reset1/1
  TienXuly/2(v'q) -> apha-beta=>dq/3(Ubeta)
  apha-beta=>dq/1(vq) -> Square1/1, PID Controller/1
  TienXuly/1(v') -> apha-beta=>dq/2(Uapha)
  2pi/1 -> Reset1/2
  wff/1 -> Sum1/2
  Reset1/1 -> Tinhtheta/2
  apha-beta=>dq/2(vd) -> Square/1
  Square/1 -> Sum/1
  Square1/1 -> Sum/2
  Sum/1 -> Sqrt/1
  Sqrt/1 -> v_dq/1
  Sum1/1 -> Low-Pass Filter (Discrete or Continuous)/1, Tinhtheta/1  "P"
  Low-Pass Filter (Discrete or Continuous)/1 -> Scope/1, omega/1  "P"

== system Simulation_18thJune/Voltage Source Inverter 3/PMW ==
  REF : Inport
  Tri_signal : Inport  Port=2
  Demux : Demux  Outputs=3
  Mux : Mux  Inputs=6
  NOT : Logic  Operator=NOT  AllPortsSameDT=off  OutDataTypeStr=boolean
  NOT1 : Logic  Operator=NOT  AllPortsSameDT=off  OutDataTypeStr=boolean
  NOT2 : Logic  Operator=NOT  AllPortsSameDT=off  OutDataTypeStr=boolean
  Relational Operator : RelationalOperator  OutDataTypeStr=boolean  RndMeth=Simplest  InputSameDT=off
  Relational Operator1 : RelationalOperator  OutDataTypeStr=boolean  RndMeth=Simplest  InputSameDT=off
  Relational Operator2 : RelationalOperator  OutDataTypeStr=boolean  RndMeth=Simplest  InputSameDT=off
  Scope : Scope
  Scope1 : Scope
  Scope2 : Scope  NumInputPorts=2
  Out1 : Outport
  wires:
  Demux/1 -> Relational Operator/1
  Tri_signal/1 -> Relational Operator1/2, Relational Operator/2, Relational Operator2/2
  Demux/2 -> Relational Operator1/1
  Demux/3 -> Relational Operator2/1
  REF/1 -> Scope1/1, Demux/1
  Relational Operator/1 -> Scope2/1, Mux/1, NOT/1
  NOT/1 -> Scope2/2, Mux/2
  Relational Operator1/1 -> NOT1/1, Mux/3
  NOT1/1 -> Mux/4
  Relational Operator2/1 -> Mux/5, NOT2/1
  NOT2/1 -> Mux/6
  Mux/1 -> Scope/1, Out1/1

== system Simulation_18thJune/Voltage Source Inverter 3/PQ calculator ==
  Vod : Inport
  Voq : Inport  Port=2
  Iod : Inport  Port=3
  Ioq : Inport  Port=4
  Product{,1..3} (4 alike) : Product
  Scope : Scope
  Sum10 : Sum  Inputs=|++
  Sum11 : Sum  Inputs=|+-
  p_hat : Outport
  q_hat : Outport  Port=2
  wires:
  Product3/1 -> Sum11/2
  Product1/1 -> Sum10/2
  Voq/1 -> Product3/1, Product1/1
  Iod/1 -> Product/2, Product3/2
  Product2/1 -> Sum11/1
  Ioq/1 -> Product1/2, Product2/2
  Product/1 -> Sum10/1
  Vod/1 -> Scope/1, Product/1, Product2/1
  Sum11/1 -> q_hat/1  "q_hat"
  Sum10/1 -> p_hat/1  "p_hat"

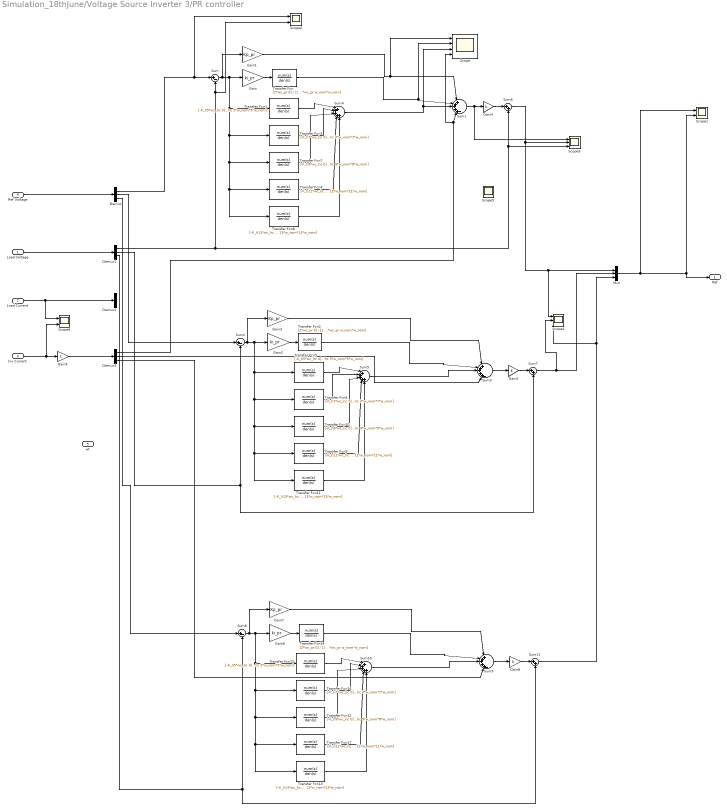
== system Simulation_18thJune/Voltage Source Inverter 3/PR controller ==
  Load Voltage : Inport
  Load Current : Inport  Port=2
  Inv Current : Inport  Port=3
  Ref Voltage : Inport  Port=4
  wt : Inport  Port=5
  Demux{,1..3} (4 alike) : Demux  Outputs=3
  Gain : Gain  Gain=ki_pr
  Gain1 : Gain  Gain=Kp_pr
  Gain2 : Gain  Gain=ki_pr
  Gain3 : Gain  Gain=Kp_pr
  Gain4 : Gain  Gain=k
  Gain5 : Gain  Gain=k
  Gain6 : Gain  Gain=ki_pr
  Gain7 : Gain  Gain=Kp_pr
  Gain8 : Gain  Gain=k
  Gain9 : Gain
  Mux : Mux  Inputs=3
  Scope : Scope  NumInputPorts=4
  Scope{1..2,5..6} (4 alike) : Scope  NumInputPorts=2
  Scope3 : Scope  NumInputPorts=3
  Scope4 : Scope  NumInputPorts=3
  Sum : Sum  Inputs=|+-
  Sum1 : Sum  Inputs=|+++++-
  Sum10 : Sum  Inputs=|+++++
  Sum11 : Sum  Inputs=|++
  Sum2 : Sum  Inputs=|+-
  Sum3 : Sum  Inputs=|+++++-
  Sum4 : Sum  Inputs=|+++++
  Sum5 : Sum  Inputs=|+++++
  Sum6 : Sum  Inputs=|++
  Sum7 : Sum  Inputs=|++
  Sum8 : Sum  Inputs=|+-
  Sum9 : Sum  Inputs=|+++++-
  Transfer Fcn : TransferFcn  Numerator=[2*wc_pr 0]  Denominator=[1 2*wc_pr*wc_pr w_nom*w_nom]
  Transfer Fcn1 : TransferFcn  Numerator=[-K_h5*wc_hc 0]  Denominator=[1 2*wc_hc 5*w_nom*5*w_nom]
  Transfer Fcn10 : TransferFcn  Numerator=[-K_h9*wc_hc 0]  Denominator=[1 2*wc_hc 9*w_nom*9*w_nom]
  Transfer Fcn11 : TransferFcn  Numerator=[-K_h13*wc_hc 0]  Denominator=[1 2*wc_hc 13*w_nom*13*w_nom]
  Transfer Fcn12 : TransferFcn  Numerator=[-K_h9*wc_hc 0]  Denominator=[1 2*wc_hc 9*w_nom*9*w_nom]
  Transfer Fcn13 : TransferFcn  Numerator=[-K_h13*wc_hc 0]  Denominator=[1 2*wc_hc 13*w_nom*13*w_nom]
  Transfer Fcn14 : TransferFcn  Numerator=[2*wc_pr 0]  Denominator=[1 2*wc_pr*wc_pr w_nom*w_nom]
  Transfer Fcn15 : TransferFcn  Numerator=[-K_h5*wc_hc 0]  Denominator=[1 2*wc_hc 5*w_nom*5*w_nom]
  Transfer Fcn16 : TransferFcn  Numerator=[-K_h7*wc_hc 0]  Denominator=[1 2*wc_hc 7*w_nom*7*w_nom]
  Transfer Fcn17 : TransferFcn  Numerator=[-K_h11*wc_hc 0]  Denominator=[1 2*wc_hc 11*w_nom*11*w_nom]
  Transfer Fcn2 : TransferFcn  Numerator=[2*wc_pr 0]  Denominator=[1 2*wc_pr*wc_pr w_nom*w_nom]
  Transfer Fcn3 : TransferFcn  Numerator=[-K_h7*wc_hc 0]  Denominator=[1 2*wc_hc 7*w_nom*7*w_nom]
  Transfer Fcn4 : TransferFcn  Numerator=[-K_h11*wc_hc 0]  Denominator=[1 2*wc_hc 11*w_nom*11*w_nom]
  Transfer Fcn5 : TransferFcn  Numerator=[-K_h5*wc_hc 0]  Denominator=[1 2*wc_hc 5*w_nom*5*w_nom]
  Transfer Fcn6 : TransferFcn  Numerator=[-K_h7*wc_hc 0]  Denominator=[1 2*wc_hc 7*w_nom*7*w_nom]
  Transfer Fcn7 : TransferFcn  Numerator=[-K_h9*wc_hc 0]  Denominator=[1 2*wc_hc 9*w_nom*9*w_nom]
  Transfer Fcn8 : TransferFcn  Numerator=[-K_h13*wc_hc 0]  Denominator=[1 2*wc_hc 13*w_nom*13*w_nom]
  Transfer Fcn9 : TransferFcn  Numerator=[-K_h11*wc_hc 0]  Denominator=[1 2*wc_hc 11*w_nom*11*w_nom]
  Ref : Outport
  wires:
  Ref Voltage/1 -> Demux/1
  Sum/1 -> Gain1/1, Transfer Fcn8/1, Transfer Fcn4/1, Transfer Fcn7/1, Transfer Fcn3/1, Transfer Fcn1/1, Gain/1
  Gain/1 -> Transfer Fcn/1
  Gain1/1 -> Scope/1, Sum1/1
  Transfer Fcn/1 -> Scope/2, Sum1/2
  Mux/1 -> Ref/1, Scope1/2, Scope1/1
  Sum4/1 -> Scope/3, Sum1/3
  Transfer Fcn1/1 -> Sum4/1
  Transfer Fcn3/1 -> Sum4/2
  Transfer Fcn7/1 -> Sum4/3
  Transfer Fcn4/1 -> Sum4/4
  Transfer Fcn8/1 -> Sum4/5
  Load Voltage/1 -> Demux1/1
  Inv Current/1 -> Scope6/2, Gain9/1
  Demux/1 -> Scope2/1, Sum/1
  Demux1/1 -> Sum6/2, Scope3/3, Scope2/2, Sum/2
  Demux3/1 -> Scope/4, Sum1/5
  Sum1/1 -> Scope3/1, Gain4/1
  Gain4/1 -> Sum6/1
  Sum6/1 -> Scope4/1, Mux/1, Scope3/2
  Demux1/2 -> Sum7/2, Sum2/2
  Transfer Fcn9/1 -> Sum5/4
  Sum5/1 -> Sum3/3
  Transfer Fcn6/1 -> Sum5/2
  Transfer Fcn5/1 -> Sum5/1
  Transfer Fcn11/1 -> Sum5/5
  Transfer Fcn10/1 -> Sum5/3
  Gain5/1 -> Sum7/1
  Gain3/1 -> Sum3/1
  Demux/2 -> Sum2/1
  Sum3/1 -> Gain5/1
  Sum2/1 -> Gain3/1, Transfer Fcn11/1, Transfer Fcn9/1, Transfer Fcn10/1, Transfer Fcn6/1, Transfer Fcn5/1, Gain2/1
  Transfer Fcn2/1 -> Sum3/2
  Gain2/1 -> Transfer Fcn2/1
  Sum7/1 -> Scope4/2, Mux/2
  Demux1/3 -> Sum11/2, Sum8/2
  Gain6/1 -> Transfer Fcn14/1
  Sum8/1 -> Gain7/1, Transfer Fcn13/1, Transfer Fcn17/1, Transfer Fcn12/1, Transfer Fcn16/1, Transfer Fcn15/1, Gain6/1
  Gain8/1 -> Sum11/1
  Sum9/1 -> Gain8/1
  Transfer Fcn13/1 -> Sum10/5
  Transfer Fcn12/1 -> Sum10/3
  Gain7/1 -> Sum9/1
  Transfer Fcn15/1 -> Sum10/1
  Transfer Fcn16/1 -> Sum10/2
  Transfer Fcn17/1 -> Sum10/4
  Sum11/1 -> Scope4/3, Mux/3
  Sum10/1 -> Sum9/3
  Demux/3 -> Sum8/1
  Transfer Fcn14/1 -> Sum9/2
  Demux3/2 -> Sum3/5
  Demux3/3 -> Sum9/5
  Load Current/1 -> Scope6/1, Demux2/1
  Gain9/1 -> Demux3/1

== system Simulation_18thJune/Voltage Source Inverter 3/dq converter ==
  Vodq : Inport
  Iodq : Inport  Port=2
  Ildq : Inport  Port=3
  wt : Inport  Port=4
  Scope : Scope
  Scope1 : Scope
  Subsystem : Subsystem
  Subsystem1 : Subsystem
  Subsystem2 : Subsystem
  Vod : Outport
  Voq : Outport  Port=2
  Iod : Outport  Port=3
  Ioq : Outport  Port=4
  Ild : Outport  Port=5
  Ilq : Outport  Port=6
  wires:
  Subsystem/1(Out1) -> Scope/1, Vod/1  "Vod"
  Subsystem1/1(Out1) -> Iod/1  "Iod"
  Subsystem/2(Out2) -> Voq/1  "Voq"
  wt/1 -> Subsystem2/2(wt), Subsystem1/2(wt), Subsystem/2(wt)
  Subsystem1/2(Out2) -> Ioq/1  "Ioq"
  Iodq/1 -> Subsystem1/1(abc)
  Subsystem2/2(Out2) -> Ilq/1  "Ilq"
  Ildq/1 -> Subsystem2/1(abc)
  Vodq/1 -> Subsystem/1(abc)
  Subsystem2/1(Out1) -> Scope1/1, Ild/1  "Vod"

== system Simulation_18thJune/Voltage Source Inverter 4/3to2 3 ==
  "single " : Inport
  "wt " : Inport  Port=2
  Add1 : Sum  Inputs=+++
  Constant2 : Constant  Value=2*pi/3
  Constant3 : Constant  Value=4*pi/3
  Constant4 : Constant  Value=exp(i*2*pi/3)
  Constant5 : Constant  Value=2/3
  Cos : Trigonometry  Operator=cos
  Cos1 : Trigonometry  Operator=cos
  Cos2 : Trigonometry  Operator=cos
  Math Function1 : Math  Operator=square  SignedPower=on
  Mux : Mux  Inputs=3
  Product{3..8} (6 alike) : Product  RndMeth=Zero
  Scope : Scope  NumInputPorts=3
  Sum : Sum  Inputs=|++
  Sum1 : Sum  Inputs=|++
  threePhase : Outport  VectorParamsAs1DForOutWhenUnconnected=off
  wires:
  "single "/1 -> Product5/1, Product4/1, Product3/1
  Cos/1 -> Product3/2
  Constant2/1 -> Sum/2
  Sum/1 -> Cos1/1
  Cos1/1 -> Product4/2
  "wt "/1 -> Sum1/1, Sum/1, Cos/1
  Constant3/1 -> Sum1/2
  Sum1/1 -> Cos2/1
  Cos2/1 -> Product5/2
  Constant4/1 -> Product7/1, Math Function1/1
  Product7/1 -> Add1/2
  Add1/1 -> Product6/1
  Product8/1 -> Add1/3
  Product5/1 -> Scope/3, Mux/3, Product8/2
  Product3/1 -> Scope/1, Mux/1, Add1/1
  Constant5/1 -> Product6/2
  Product4/1 -> Scope/2, Mux/2, Product7/2
  Math Function1/1 -> Product8/1
  Mux/1 -> threePhase/1

== system Simulation_18thJune/Voltage Source Inverter 4/Droop for secondary control2 ==
  P : Inport
  w_nom : Inport  Port=2
  V_nom : Inport  Port=3
  Q : Inport  Port=4
  Gain4 : Gain  Gain=n_q
  Gain5 : Gain  Gain=m_p
  Integrator : Integrator  WrapState=on  WrappedStateUpperValue=2*pi  WrappedStateLowerValue=0
  Sum1 : Sum  Inputs=|+-
  Sum2 : Sum  Inputs=|+-
  Vref : Outport
  wt : Outport  Port=2
  wo : Outport  Port=3
  wires:
  P/1 -> Gain5/1
  w_nom/1 -> Sum2/1
  Gain5/1 -> Sum2/2
  Sum2/1 -> wo/1, Integrator/1  "w"
  Integrator/1 -> wt/1
  V_nom/1 -> Sum1/1  "Vod_s"
  Gain4/1 -> Sum1/2
  Q/1 -> Gain4/1
  Sum1/1 -> Vref/1  "Vod_s"

== system Simulation_18thJune/Voltage Source Inverter 4/Low-pass filter ==
  p_hat : Inport
  q_hat : Inport  Port=2
  Low-Pass Filter (Discrete or Continuous) : eeGeneralControl/Low-Pass Filter (Discrete or Continuous)  K=1  T=lo_co  B=inf  A=-inf  init_option=Inherited from block input  x0=0  Ts=-1
  Low-Pass Filter (Discrete or Continuous)1 : eeGeneralControl/Low-Pass Filter (Discrete or Continuous)  K=1  T=lo_co  B=inf  A=-inf  init_option=Inherited from block input  x0=0  Ts=-1
  P : Outport
  Q : Outport  Port=2
  wires:
  q_hat/1 -> Low-Pass Filter (Discrete or Continuous)1/1
  Low-Pass Filter (Discrete or Continuous)1/1 -> Q/1  "Q"
  Low-Pass Filter (Discrete or Continuous)/1 -> P/1  "P"
  p_hat/1 -> Low-Pass Filter (Discrete or Continuous)/1

== system Simulation_18thJune/Voltage Source Inverter 4/PLL_1p1 ==
  v : Inport
  2pi : Constant  Value=2*pi
  Low-Pass Filter (Discrete or Continuous) : eeGeneralControl/Low-Pass Filter (Discrete or Continuous)  K=1  T=lo_co  B=inf  A=-inf  init_option=Inherited from block input  x0=0  Ts=-1
  PID Controller : slpidlib/PID Controller  Controller=PI  Form=Parallel  TimeDomain=Continuous-time  UseExternalTs=off  SampleTime=-1  IntegratorMethod=Forward Euler  FilterMethod=Forward Euler  ControllerParametersSource=internal  P=100.15925  I=9869  UseKiTs=off  D=0  N=100  UseFilter=on  TunerSelectOption=Transfer Function Based (PID Tuner App)  InitialConditionSource=internal  InitialConditionForIntegrator=0  InitialConditionForFilter=0  DifferentiatorICPrevScaledInput=0  ExternalReset=none  TrackingMode=off  Kt=1  LimitOutput=off  SatLimitsSource=internal  UpperSaturationLimit=inf  LowerSaturationLimit=-inf  LinearizeAsGain=off  AntiWindupMode=none  Kb=1  LimitIntegrator=off  UpperIntegratorSaturationLimit=inf  LowerIntegratorSaturationLimit=-inf  POutMin=[]  POutMax=[]  IOutMin=[]  IOutMax=[]  DOutMin=[]  DOutMax=[]  NOutMin=[]  NOutMax=[]  SumOutMin=[]  SumOutMax=[]  SaturationOutMin=[]  SaturationOutMax=[]  PParamMin=[]  PParamMax=[]  IParamMin=[]  IParamMax=[]  DParamMin=[]  DParamMax=[]  NParamMin=[]  NParamMax=[]  KbParamMin=[]  KbParamMax=[]  KtParamMin=[]  KtParamMax=[]  KbOutMin=[]  KbOutMax=[]  KtOutMin=[]  KtOutMax=[]  IntegratorOutMin=[]  IntegratorOutMax=[]  FilterOutMin=[]  FilterOutMax=[]  SumI1OutMin=[]  SumI1OutMax=[]  SumI2OutMin=[]  SumI2OutMax=[]  SumI3OutMin=[]  SumI3OutMax=[]  SumI4OutMin=[]  SumI4OutMax=[]  SumDOutMin=[]  SumDOutMax=[]  DifferentiatorOutMin=[]  DifferentiatorOutMax=[]  FilterDiffOutCoefMin=[]  FilterDiffOutCoefMax=[]  ReciprocalOutMin=[]  ReciprocalOutMax=[]  SumDenOutMin=[]  SumDenOutMax=[]  SumNumOutMin=[]  SumNumOutMax=[]  DivideOutMin=[]  DivideOutMax=[]  UdiffTsProdOutMin=[]  UdiffTsProdOutMax=[]  NTsProdOutMin=[]  NTsProdOutMax=[]  UintegralTsProdOutMin=[]  UintegralTsProdOutMax=[]  UngainTsProdOutMin=[]  UngainTsProdOutMax=[]  ClampingZeroOutDataTypeStr=Inherit: Inherit via back propagation  ClampingZeroOutMin=[]  ClampingZeroOutMax=[]  FilterDenConstantOutDataTypeStr=Inherit: Inherit via back propagation  FilterDenConstantOutMin=[]  FilterDenConstantOutMax=[]  PCopyOutDataTypeStr=Inherit: Inherit via back propagation  PCopyOutMin=[]  PCopyOutMax=[]  NCopyOutDataTypeStr=Inherit: Inherit via back propagation  NCopyOutMin=[]  NCopyOutMax=[]  IntegratorContinuousStateAttributes=''  IntegratorStateMustResolveToSignalObject=off  IntegratorRTWStateStorageClass=Auto  FilterContinuousStateAttributes=''  FilterStateMustResolveToSignalObject=off  FilterRTWStateStorageClass=Auto  ParallelPVariant=InternalParameters  IdealPVariant=Disabled  IVariant=InternalParameters  DVariant=Disabled  IntegratorVariant=Continuous  SatVariant=Disabled  AWVariant=Passthrough  PCopyVariant=Disabled  TRVariant=Disabled  FdbkBlocksVariant=Forward  IdealPFdbkVariant=Disabled  SatFdbkVariant=Disabled  DerivativeFilterVariant=Disabled  NVariant=Disabled  NCopyVariant=Disabled_SignalSpec  FilterICVariant=Disabled  IntegratorICVariant=InternalICs  ExternalResetVariant=Disabled  TRSumVariant=Passthrough  SumFdbkVariant=Disabled  SumVariant=Sum_PI  TsampFilterVariant=InternalTs  TsampNgainVariant=Passthrough  TsampIntegralVariant=Passthrough  ExternalSaturationOutDataTypeStr=Inherit: Same as second input
  Reset1 : RelationalOperator  OutDataTypeStr=boolean  InputSameDT=off
  Scope : Scope
  Sqrt : Sqrt
  Square : Math  Operator=square
  Square1 : Math  Operator=square
  Sum : Sum  Inputs=|++
  Sum1 : Sum  Inputs=|++
  TienXuly : Subsystem  mask{k=0.5, fc1=50, fc2=10}
      mask prompts: k "he so k"; fc1 "Tan so cat cua bo loc bac 2"; fc2 "Tan so cat cua bo loc thong thap"
  Tinhtheta : Integrator  ExternalReset=rising  UpperSaturationLimit=2*pi
  apha-beta=>dq : Subsystem
  wff : Constant  Value=50*2*pi
  v_dq : Outport
  omega : Outport  Port=2
  wires:
  PID Controller/1 -> Sum1/1
  v/1 -> TienXuly/1(v)
  Tinhtheta/1 -> apha-beta=>dq/1(Theta), Reset1/1
  TienXuly/2(v'q) -> apha-beta=>dq/3(Ubeta)
  apha-beta=>dq/1(vq) -> Square1/1, PID Controller/1
  TienXuly/1(v') -> apha-beta=>dq/2(Uapha)
  2pi/1 -> Reset1/2
  wff/1 -> Sum1/2
  Reset1/1 -> Tinhtheta/2
  apha-beta=>dq/2(vd) -> Square/1
  Square/1 -> Sum/1
  Square1/1 -> Sum/2
  Sum/1 -> Sqrt/1
  Sqrt/1 -> v_dq/1
  Sum1/1 -> Low-Pass Filter (Discrete or Continuous)/1, Tinhtheta/1  "P"
  Low-Pass Filter (Discrete or Continuous)/1 -> Scope/1, omega/1  "P"

== system Simulation_18thJune/Voltage Source Inverter 4/PLL_1p2 ==
  v : Inport
  2pi : Constant  Value=2*pi
  Low-Pass Filter (Discrete or Continuous) : eeGeneralControl/Low-Pass Filter (Discrete or Continuous)  K=1  T=lo_co  B=inf  A=-inf  init_option=Inherited from block input  x0=0  Ts=-1
  PID Controller : slpidlib/PID Controller  Controller=PI  Form=Parallel  TimeDomain=Continuous-time  UseExternalTs=off  SampleTime=-1  IntegratorMethod=Forward Euler  FilterMethod=Forward Euler  ControllerParametersSource=internal  P=100.15925  I=9869  UseKiTs=off  D=0  N=100  UseFilter=on  TunerSelectOption=Transfer Function Based (PID Tuner App)  InitialConditionSource=internal  InitialConditionForIntegrator=0  InitialConditionForFilter=0  DifferentiatorICPrevScaledInput=0  ExternalReset=none  TrackingMode=off  Kt=1  LimitOutput=off  SatLimitsSource=internal  UpperSaturationLimit=inf  LowerSaturationLimit=-inf  LinearizeAsGain=off  AntiWindupMode=none  Kb=1  LimitIntegrator=off  UpperIntegratorSaturationLimit=inf  LowerIntegratorSaturationLimit=-inf  POutMin=[]  POutMax=[]  IOutMin=[]  IOutMax=[]  DOutMin=[]  DOutMax=[]  NOutMin=[]  NOutMax=[]  SumOutMin=[]  SumOutMax=[]  SaturationOutMin=[]  SaturationOutMax=[]  PParamMin=[]  PParamMax=[]  IParamMin=[]  IParamMax=[]  DParamMin=[]  DParamMax=[]  NParamMin=[]  NParamMax=[]  KbParamMin=[]  KbParamMax=[]  KtParamMin=[]  KtParamMax=[]  KbOutMin=[]  KbOutMax=[]  KtOutMin=[]  KtOutMax=[]  IntegratorOutMin=[]  IntegratorOutMax=[]  FilterOutMin=[]  FilterOutMax=[]  SumI1OutMin=[]  SumI1OutMax=[]  SumI2OutMin=[]  SumI2OutMax=[]  SumI3OutMin=[]  SumI3OutMax=[]  SumI4OutMin=[]  SumI4OutMax=[]  SumDOutMin=[]  SumDOutMax=[]  DifferentiatorOutMin=[]  DifferentiatorOutMax=[]  FilterDiffOutCoefMin=[]  FilterDiffOutCoefMax=[]  ReciprocalOutMin=[]  ReciprocalOutMax=[]  SumDenOutMin=[]  SumDenOutMax=[]  SumNumOutMin=[]  SumNumOutMax=[]  DivideOutMin=[]  DivideOutMax=[]  UdiffTsProdOutMin=[]  UdiffTsProdOutMax=[]  NTsProdOutMin=[]  NTsProdOutMax=[]  UintegralTsProdOutMin=[]  UintegralTsProdOutMax=[]  UngainTsProdOutMin=[]  UngainTsProdOutMax=[]  ClampingZeroOutDataTypeStr=Inherit: Inherit via back propagation  ClampingZeroOutMin=[]  ClampingZeroOutMax=[]  FilterDenConstantOutDataTypeStr=Inherit: Inherit via back propagation  FilterDenConstantOutMin=[]  FilterDenConstantOutMax=[]  PCopyOutDataTypeStr=Inherit: Inherit via back propagation  PCopyOutMin=[]  PCopyOutMax=[]  NCopyOutDataTypeStr=Inherit: Inherit via back propagation  NCopyOutMin=[]  NCopyOutMax=[]  IntegratorContinuousStateAttributes=''  IntegratorStateMustResolveToSignalObject=off  IntegratorRTWStateStorageClass=Auto  FilterContinuousStateAttributes=''  FilterStateMustResolveToSignalObject=off  FilterRTWStateStorageClass=Auto  ParallelPVariant=InternalParameters  IdealPVariant=Disabled  IVariant=InternalParameters  DVariant=Disabled  IntegratorVariant=Continuous  SatVariant=Disabled  AWVariant=Passthrough  PCopyVariant=Disabled  TRVariant=Disabled  FdbkBlocksVariant=Forward  IdealPFdbkVariant=Disabled  SatFdbkVariant=Disabled  DerivativeFilterVariant=Disabled  NVariant=Disabled  NCopyVariant=Disabled_SignalSpec  FilterICVariant=Disabled  IntegratorICVariant=InternalICs  ExternalResetVariant=Disabled  TRSumVariant=Passthrough  SumFdbkVariant=Disabled  SumVariant=Sum_PI  TsampFilterVariant=InternalTs  TsampNgainVariant=Passthrough  TsampIntegralVariant=Passthrough  ExternalSaturationOutDataTypeStr=Inherit: Same as second input
  Reset1 : RelationalOperator  OutDataTypeStr=boolean  InputSameDT=off
  Scope : Scope
  Sqrt : Sqrt
  Square : Math  Operator=square
  Square1 : Math  Operator=square
  Sum : Sum  Inputs=|++
  Sum1 : Sum  Inputs=|++
  TienXuly : Subsystem  mask{k=0.5, fc1=50, fc2=10}
      mask prompts: k "he so k"; fc1 "Tan so cat cua bo loc bac 2"; fc2 "Tan so cat cua bo loc thong thap"
  Tinhtheta : Integrator  ExternalReset=rising  UpperSaturationLimit=2*pi
  apha-beta=>dq : Subsystem
  wff : Constant  Value=50*2*pi
  v_dq : Outport
  omega : Outport  Port=2
  wires:
  PID Controller/1 -> Sum1/1
  v/1 -> TienXuly/1(v)
  Tinhtheta/1 -> apha-beta=>dq/1(Theta), Reset1/1
  TienXuly/2(v'q) -> apha-beta=>dq/3(Ubeta)
  apha-beta=>dq/1(vq) -> Square1/1, PID Controller/1
  TienXuly/1(v') -> apha-beta=>dq/2(Uapha)
  2pi/1 -> Reset1/2
  wff/1 -> Sum1/2
  Reset1/1 -> Tinhtheta/2
  apha-beta=>dq/2(vd) -> Square/1
  Square/1 -> Sum/1
  Square1/1 -> Sum/2
  Sum/1 -> Sqrt/1
  Sqrt/1 -> v_dq/1
  Sum1/1 -> Low-Pass Filter (Discrete or Continuous)/1, Tinhtheta/1  "P"
  Low-Pass Filter (Discrete or Continuous)/1 -> Scope/1, omega/1  "P"

== system Simulation_18thJune/Voltage Source Inverter 4/PMW ==
  REF : Inport
  Tri_signal : Inport  Port=2
  Demux : Demux  Outputs=3
  Mux : Mux  Inputs=6
  NOT : Logic  Operator=NOT  AllPortsSameDT=off  OutDataTypeStr=boolean
  NOT1 : Logic  Operator=NOT  AllPortsSameDT=off  OutDataTypeStr=boolean
  NOT2 : Logic  Operator=NOT  AllPortsSameDT=off  OutDataTypeStr=boolean
  Relational Operator : RelationalOperator  OutDataTypeStr=boolean  RndMeth=Simplest  InputSameDT=off
  Relational Operator1 : RelationalOperator  OutDataTypeStr=boolean  RndMeth=Simplest  InputSameDT=off
  Relational Operator2 : RelationalOperator  OutDataTypeStr=boolean  RndMeth=Simplest  InputSameDT=off
  Scope : Scope
  Scope1 : Scope
  Scope2 : Scope  NumInputPorts=2
  Out1 : Outport
  wires:
  Demux/1 -> Relational Operator/1
  Tri_signal/1 -> Relational Operator1/2, Relational Operator/2, Relational Operator2/2
  Demux/2 -> Relational Operator1/1
  Demux/3 -> Relational Operator2/1
  REF/1 -> Scope1/1, Demux/1
  Relational Operator/1 -> Scope2/1, Mux/1, NOT/1
  NOT/1 -> Scope2/2, Mux/2
  Relational Operator1/1 -> NOT1/1, Mux/3
  NOT1/1 -> Mux/4
  Relational Operator2/1 -> Mux/5, NOT2/1
  NOT2/1 -> Mux/6
  Mux/1 -> Scope/1, Out1/1
